simulink model "Sim22"  (R2019a)
settings: Solver=FixedStepAuto  StartTime=0.0  StopTime=10.0  FixedStep=0.0001  RelTol=1e-3
settings Model: Creator=fbleo  LastModifiedBy=fbleo

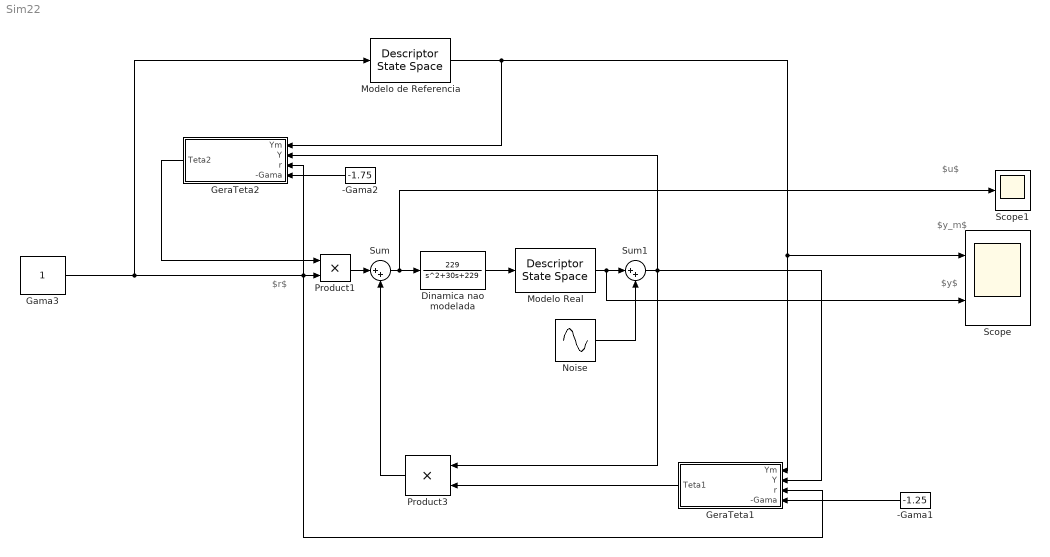
== system Sim22 ==
  note: $u$
  note: $r$
  note: $y$
  note: $y_m$
  -Gama1 : Constant  Value=-1.25
  -Gama2 : Constant  Value=-1.75
  Dinamica nao modelada : TransferFcn  Numerator=[229]  Denominator=[1 30 229]
  Gama3 : Constant
  GeraTeta1 : Subsystem
  GeraTeta2 : Subsystem
  Modelo Real : DescriptorStateSpace  A=-1  B=2  D=0  InitialCondition=0.5
  Modelo de Referencia : DescriptorStateSpace  A=-3  B=3  D=0  InitialCondition=0
  Noise : Sin  Amplitude=0.1  Frequency=16.1  SampleTime=0
  Product1 : Product
  Product3 : Product
  Scope : Scope  NumInputPorts=2
  Scope1 : Scope
  Sum : Sum  Inputs=|++
  Sum1 : Sum  Inputs=|++
  wires:
  Modelo de Referencia/1 -> GeraTeta2/1(Ym), GeraTeta1/1(Ym), Scope/1
  Gama3/1 -> GeraTeta1/3(r), GeraTeta2/3(r), Product1/2, Modelo de Referencia/1
  Sum1/1 -> GeraTeta2/2(Y), GeraTeta1/2(Y), Product3/1
  Noise/1 -> Sum1/2
  Modelo Real/1 -> Scope/2, Sum1/1
  GeraTeta1/1("Teta1 ") -> Product3/2
  Sum/1 -> Scope1/1, Dinamica nao modelada/1
  Dinamica nao modelada/1 -> Modelo Real/1
  -Gama1/1 -> GeraTeta1/4(-Gama)
  Product3/1 -> Sum/2
  -Gama2/1 -> GeraTeta2/4(-Gama)
  Product1/1 -> Sum/1
  GeraTeta2/1(Teta2) -> Product1/1

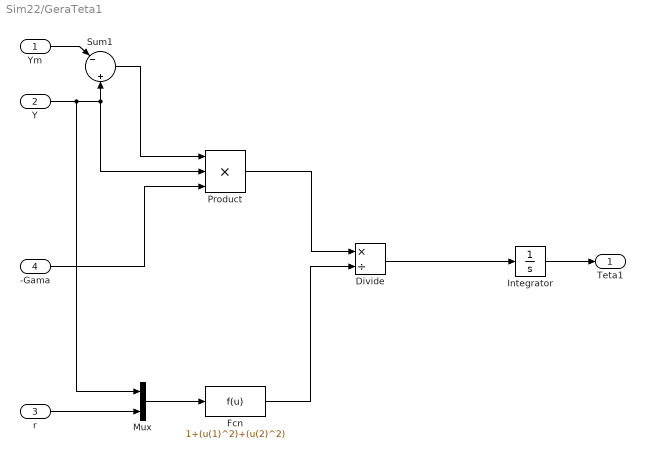
== system Sim22/GeraTeta1 ==
  Ym : Inport
  Y : Inport  Port=2
  r : Inport  Port=3
  -Gama : Inport  Port=4
  Divide : Product  Inputs=*/
  Fcn : Fcn  Expr=1+(u(1)^2)+(u(2)^2)
  Integrator : Integrator  InitialCondition=-0.65
  Mux : Mux  Inputs=2
  Product : Product  Inputs=3
  Sum1 : Sum  Inputs=|-||+
  "Teta1 " : Outport
  wires:
  Ym/1 -> Sum1/1
  Y/1 -> Mux/1, Product/2, Sum1/2
  Sum1/1 -> Product/1
  r/1 -> Mux/2
  -Gama/1 -> Product/3
  Integrator/1 -> "Teta1 "/1
  Mux/1 -> Fcn/1
  Product/1 -> Divide/1
  Fcn/1 -> Divide/2
  Divide/1 -> Integrator/1

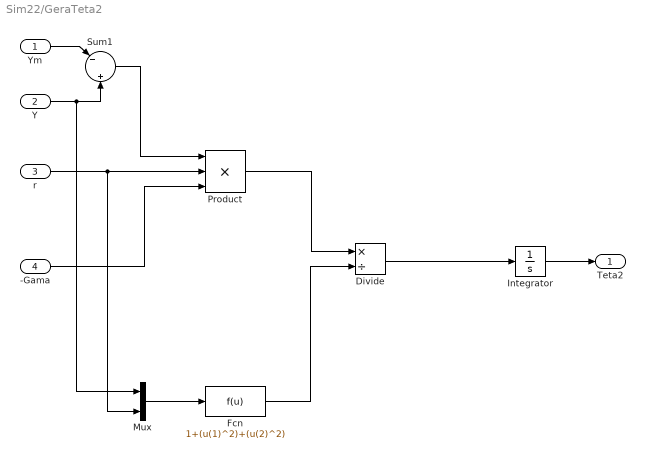
== system Sim22/GeraTeta2 ==
  Ym : Inport
  Y : Inport  Port=2
  r : Inport  Port=3
  -Gama : Inport  Port=4
  Divide : Product  Inputs=*/
  Fcn : Fcn  Expr=1+(u(1)^2)+(u(2)^2)
  Integrator : Integrator  InitialCondition=1.14
  Mux : Mux  Inputs=2
  Product : Product  Inputs=3
  Sum1 : Sum  Inputs=|-||+
  Teta2 : Outport
  wires:
  Ym/1 -> Sum1/1
  Y/1 -> Mux/1, Sum1/2
  Sum1/1 -> Product/1
  r/1 -> Mux/2, Product/2
  -Gama/1 -> Product/3
  Integrator/1 -> Teta2/1
  Mux/1 -> Fcn/1
  Product/1 -> Divide/1
  Fcn/1 -> Divide/2
  Divide/1 -> Integrator/1
